simulink library "vmc"  (R2021b)
settings: Solver=VariableStepAuto  StartTime=0.0  StopTime=10.0  RelTol=1e-3
undefined symbols (not defined in the file or in its folder): AVMC_ACCDeltaTqIGain4OVRD_X_kph, AVMC_ACCDeltaTqIGain4OVRD_Y_mps2, AVMC_ACCDeltaTqIGain_X_kph, AVMC_ACCDeltaTqIGain_Y_mps2, AVMC_ACCDeltaTqPGain_X_kph, AVMC_ACCDeltaTqPGain_Y_kph, AVMC_ACCLongSteadyCtrl_X_kph, AVMC_ADSPosGFBDeltaTq_X_kph, AVMC_ADSPosGFBDeltaTq_Y_mps2, AVMC_AggressJerkPCT4AT_X_kph, AVMC_AggressJerkPCT_X_kph, AVMC_AggressLimitPCT4AT_X_kph, AVMC_AggressLimitPCT_X_kph, AVMC_CCLongSteadyCtrl_X_kph, AVMC_DISCDeltaTqIGain_X_kph, AVMC_DISCDeltaTqIGain_Y_mps2, AVMC_DISCDeltaTqPGain_X_kph, AVMC_DISCDeltaTqPGain_Y_kph, AVMC_ESCRegenOut_X_kph, AVMC_ESCRegenOut_Y_Deg, AVMC_ESCRegenOutEnSpd_X_Deg, AVMC_ISOAccLimit_X_mps, AVMC_ISODecLimit_X_mps, AVMC_ISOJerk_X_mps, AVMC_LatESCRegenOut_X_kph, AVMC_LatESCRegenOut_Y_Deg, AVMC_LongAccDeadZone_X_kph, AVMC_LongAccFiltTsforP2_X_Gps, AVMC_MCPresBaseTq_X_bar, AVMC_MSALongSteadyCtrl_X_kph, AVMC_MSAPedalOvrd_X_kph, AVMC_MSASpdBand_X_kph, AVMC_MSATqDownEndTq_X_kph, AVMC_MSATqDownTime_X_kph, AVMC_OPDDisSlideRate_X_Deg, AVMC_OVRD2ActSR2FCMCMD_X_mps2, AVMC_PedalTqRWhlRatio_X_Nm, AVMC_PedalTqRWhlRatio_Y_gps, AVMC_PedalTqRWhlSlipGain_X_rat, AVMC_PedalTqRWhlSlipGain_Y_kph, AVMC_PedalTqRWhSTRGGain_X_deg, AVMC_PedalTqRWhSTRGGain_Y_kph, AVMC_RDCDetectTime_X_kph, AVMC_RDCDetectTime_Y_pct, AVMC_RDCEnSlideRate_X_Deg, AVMC_RearWhlTqRatio_X_Nm, AVMC_RearWhlTqRatio_Y_gps, AVMC_RearWhlTqSlipGain_X_rat, AVMC_RearWhlTqSlipGain_Y_kph, AVMC_RearWhlTqSTRGGain_X_deg, AVMC_RearWhlTqSTRGGain_Y_kph, AVMC_ReqBrkJoinDecSR_X_mps2, AVMC_SoftJerkPCT_X_kph, AVMC_SoftLimitPCT_X_kph, AVMC_StESCYaw_X_kph, AVMC_StESCYaw_Y_Deg, AVMC_StESCYawCom_X_kph, AVMC_StESCYawCom_Y_Gps, AVMC_TMSpdBaseTq_X_rpm, AVMC_VehHoldDecCtrlTime2_X_kph ... (+411)
libraries: hcu_lib x108, simulink x82, tqr x1, simulink_extras x1
(part 8 of 14)

== system vmc/VMC/VMC/APS function/Signal Rounting1 ==
  VINP_SCPSystemMode_enum : Inport
  VVMC_APSActive_flg : Inport  Port=2
  VVMC_ADASActive_flg : Inport  Port=3
  VTQD_GearActualPosn_enum : Inport  Port=4
  VVMC_CAASActive_flg : Inport  Port=5
  VTQD_APSStaSys_enum : Inport  Port=6
  VTQD_APSDecReqA_flg : Inport  Port=7
  VTQD_APSDecReq_mps2 : Inport  Port=8
  VTQD_APSReq_enum : Inport  Port=9
  VINP_APSStaSystem_enum : Inport  Port=10
  VINP_APSDecReqA_flg : Inport  Port=11
  VINP_APSDecReq_mps2 : Inport  Port=12
  VINP_APSReq_enum : Inport  Port=13
  VVMC_SetACCDisableAPS_flg : Inport  Port=14
  Signal Determination VINP_APSDecReqAtest_flg : Subsystem
  Signal Determination VINP_APSDecReqtest_mps2 : Subsystem
  Signal Determination VINP_APSReqtest_enum : Subsystem
  Signal Determination VINP_APSStaSystemtest_enum : Subsystem
  Switch{,1..3} (4 alike) : Switch  Criteria=u2 > Threshold
  VVMC_APSStaSys_enum : Outport
  VVMC_APSDecReqA_flg : Outport  Port=2
  VVMC_APSDecReq_mps2 : Outport  Port=3
  VVMC_APSReq_enum : Outport  Port=4
  wires:
  [VINP_SCPSystemMode_enum] -> Signal Determination VINP_APSDecReqtest_mps2/3(VINP_SCPSystemMode_enum)
  Signal Determination VINP_APSDecReqAtest_flg/1(SignalOutp) -> VVMC_APSDecReqA_flg/1  "VVMC_APSDecReqA_flg"
  Signal Determination VINP_APSReqtest_enum/1(SignalOutp) -> VVMC_APSReq_enum/1  "VVMC_APSReq_enum"
  [VINP_SCPSystemMode_enum] -> Signal Determination VINP_APSReqtest_enum/3(VINP_SCPSystemMode_enum)
  Signal Determination VINP_APSStaSystemtest_enum/1(SignalOutp) -> VVMC_APSStaSys_enum/1  "VVMC_APSStaSys_enum"
  [VINP_SCPSystemMode_enum] -> Signal Determination VINP_APSDecReqAtest_flg/3(VINP_SCPSystemMode_enum)
  Signal Determination VINP_APSDecReqtest_mps2/1(SignalOutp) -> VVMC_APSDecReq_mps2/1  "VVMC_APSDecReq_mps2"
  VINP_SCPSystemMode_enum/1 -> [VINP_SCPSystemMode_enum]
  VVMC_APSActive_flg/1 -> [VVMC_APSActive_flg]
  VVMC_ADASActive_flg/1 -> [VVMC_ADASActive_flg]
  [VVMC_APSActive_flg] -> Signal Determination VINP_APSStaSystemtest_enum/4(VVMC_APSActive_flg)
  [VVMC_ADASActive_flg] -> Signal Determination VINP_APSStaSystemtest_enum/5(VVMC_ADASActive_flg)
  [VVMC_APSActive_flg] -> Signal Determination VINP_APSDecReqAtest_flg/4(VVMC_APSActive_flg)
  [VVMC_ADASActive_flg] -> Signal Determination VINP_APSDecReqAtest_flg/5(VVMC_ADASActive_flg)
  [VVMC_APSActive_flg] -> Signal Determination VINP_APSDecReqtest_mps2/4(VVMC_APSActive_flg)
  [VVMC_ADASActive_flg] -> Signal Determination VINP_APSDecReqtest_mps2/5(VVMC_ADASActive_flg)
  [VVMC_APSActive_flg] -> Signal Determination VINP_APSReqtest_enum/4(VVMC_APSActive_flg)
  [VVMC_ADASActive_flg] -> Signal Determination VINP_APSReqtest_enum/5(VVMC_ADASActive_flg)
  VTQD_GearActualPosn_enum/1 -> [VTQD_GearActualPosn_enum]
  [VTQD_GearActualPosn_enum] -> Signal Determination VINP_APSStaSystemtest_enum/6(VTQD_GearActualPosn_enum)
  [VINP_SCPSystemMode_enum] -> Signal Determination VINP_APSStaSystemtest_enum/3(VINP_SCPSystemMode_enum)
  [VINP_APSReq_enum] -> Signal Determination VINP_APSReqtest_enum/1(SignalInput1)
  VVMC_CAASActive_flg/1 -> [VVMC_CAASActive_flg]
  [VVMC_CAASActive_flg] -> Signal Determination VINP_APSStaSystemtest_enum/7(VVMC_CAASActive_flg)
  [VVMC_CAASActive_flg] -> Signal Determination VINP_APSDecReqAtest_flg/6(VVMC_CAASActive_flg)
  [VVMC_CAASActive_flg] -> Signal Determination VINP_APSDecReqtest_mps2/6(VVMC_CAASActive_flg)
  [VVMC_CAASActive_flg] -> Signal Determination VINP_APSReqtest_enum/6(VVMC_CAASActive_flg)
  VTQD_APSDecReq_mps2/1 -> [VTQD_APSDecReq_mps2]
  VTQD_APSReq_enum/1 -> [VTQD_APSReq_enum]
  VTQD_APSDecReqA_flg/1 -> [VTQD_APSDecReqA_flg]
  VTQD_APSStaSys_enum/1 -> [VTQD_APSStaSys_enum]
  Switch/1 -> Signal Determination VINP_APSStaSystemtest_enum/2(SignalInput2)
  Switch1/1 -> Signal Determination VINP_APSDecReqAtest_flg/2(SignalInput2)
  Switch2/1 -> Signal Determination VINP_APSDecReqtest_mps2/2(SignalInput2)
  Switch3/1 -> Signal Determination VINP_APSReqtest_enum/2(SignalInput2)
  VINP_APSStaSystem_enum/1 -> [VINP_APSStaSystem_enum]
  VINP_APSDecReqA_flg/1 -> [VINP_APSDecReqA_flg]
  VINP_APSReq_enum/1 -> [VINP_APSReq_enum]
  VINP_APSDecReq_mps2/1 -> [VINP_APSDecReq_mps2]
  [VINP_APSDecReq_mps2] -> Signal Determination VINP_APSDecReqtest_mps2/1(SignalInput1)
  [VINP_APSDecReqA_flg] -> Signal Determination VINP_APSDecReqAtest_flg/1(SignalInput1)
  [VINP_APSStaSystem_enum] -> Signal Determination VINP_APSStaSystemtest_enum/1(SignalInput1)
  VVMC_SetACCDisableAPS_flg/1 -> [VVMC_SetACCDisableAPS_flg]
  [VVMC_SetACCDisableAPS_flg] -> Switch/2
  [VINP_APSStaSystem_enum] -> Switch/1
  [VTQD_APSStaSys_enum] -> Switch/3
  [VVMC_SetACCDisableAPS_flg] -> Switch1/2
  [VTQD_APSDecReqA_flg] -> Switch1/3
  [VINP_APSDecReqA_flg] -> Switch1/1
  [VVMC_SetACCDisableAPS_flg] -> Switch2/2
  [VTQD_APSDecReq_mps2] -> Switch2/3
  [VINP_APSDecReq_mps2] -> Switch2/1
  [VVMC_SetACCDisableAPS_flg] -> Switch3/2
  [VTQD_APSReq_enum] -> Switch3/3
  [VINP_APSReq_enum] -> Switch3/1

== system vmc/VMC/VMC/APS function/Subsystem ==
  VINP_ADASACCSta_enum : Inport
  VINP_MCPressure_bar : Inport  Port=2
  VINP_BrkSwSta_flg : Inport  Port=3
  VINP_BrkPedalPos_pct : Inport  Port=4
  VTQD_APSDecReqA_flg : Inport  Port=5
  VINP_ACCObjDist_m : Inport  Port=6
  VVMC_MeterIndSpeedForCalcu_kph : Inport  Port=7
  VINP_VehSpeed_kph : Inport  Port=8
  0 : Constant  Value=KVMC_AllowSetSpdOvrd_flg
  1 : Constant  Value=KVMC_AllowSetSpdOvrdVal_flg
  2m : Constant  Value=KVMC_NotAllowSetSpdDist_m
  6m : Constant  Value=KVMC_AllowSetSpdDist_m
  AND : Logic  Inputs=6  AllPortsSameDT=off  OutDataTypeStr=boolean
  AND1 : Logic  Operator=OR  AllPortsSameDT=off  OutDataTypeStr=boolean
  AND3 : Logic  AllPortsSameDT=off  OutDataTypeStr=boolean
  Constant1 : Constant  Value=ENUM_ADASACCSTA_ACTIVE
  Constant2 : Constant  Value=ENUM_ADASACCSTA_STANDBY
  Constant4 : Constant  Value=KVMC_APSAllowSetACCMCP_bar
  Constant5 : Constant  Value=ZERO_FLOAT
  Constant6 : Constant  Value=TRUE
  Constant7 : Constant  Value=KVMC_APSAllowSetACCPosn_pct
  NOT : Logic  Operator=NOT  AllPortsSameDT=off  OutDataTypeStr=boolean
  NOT1 : Logic  Operator=NOT  AllPortsSameDT=off  OutDataTypeStr=boolean
  Relational Operator : RelationalOperator  Operator===  OutDataTypeStr=boolean  RndMeth=Simplest
  Relational Operator1 : RelationalOperator  Operator===  OutDataTypeStr=boolean  RndMeth=Simplest
  Relational Operator{2..4,6} (4 alike) : RelationalOperator  Operator=>  OutDataTypeStr=boolean  RndMeth=Simplest
  Relational Operator5 : RelationalOperator  Operator=<=  OutDataTypeStr=boolean  RndMeth=Simplest
  SR_Latch2 : hcu_lib/Basic_Blocks/SR_Latch
  Switch : Switch  Criteria=u2 > Threshold
  Switch1 : Switch  Criteria=u2 > Threshold
  VVMC_SetACCDisableAPS_flg : Outport
  wires:
  NOT1/1 -> AND/6
  Constant6/1 -> Switch/3
  Relational Operator4/1 -> AND/5
  AND/1 -> SR_Latch2/1
  Relational Operator1/1 -> AND1/1
  Constant2/1 -> Relational Operator/2
  Relational Operator3/1 -> NOT1/1
  Constant5/1 -> Relational Operator3/2
  Relational Operator/1 -> AND/1
  AND1/1 -> SR_Latch2/2
  Switch/1 -> VVMC_SetACCDisableAPS_flg/1  "VVMC_SetACCDisableAPS_flg"
  [VINP_VehSpeed_kph] -> Relational Operator3/1
  [VINP_MCPressure_bar] -> Relational Operator2/1
  [VVMC_AllowSetSpd_flg] -> AND/2
  [VINP_BrkSwSta_flg] -> NOT/1
  VINP_BrkSwSta_flg/1 -> [VINP_BrkSwSta_flg]
  NOT/1 -> AND1/2
  Constant7/1 -> Relational Operator4/2
  Constant4/1 -> Relational Operator2/2
  [VINP_BrkPedalPos_pct] -> Relational Operator4/1
  Constant1/1 -> Relational Operator1/2
  [VINP_ADASACCSta_enum] -> Relational Operator1/1
  [VINP_ADASACCSta_enum] -> Relational Operator/1
  SR_Latch2/1 -> Switch/1
  Relational Operator2/1 -> AND/4
  6m/1 -> Relational Operator5/2
  Relational Operator6/1 -> AND3/2
  1/1 -> Switch1/1
  [VINP_ACCObjDist_m] -> Relational Operator6/1, Relational Operator5/1
  2m/1 -> Relational Operator6/2
  Relational Operator5/1 -> AND3/1
  0/1 -> Switch1/2
  Switch1/1 -> [VVMC_AllowSetSpd_flg]  "VVMC_AllowSetSpd_flg"
  AND3/1 -> Switch1/3
  VINP_ACCObjDist_m/1 -> [VINP_ACCObjDist_m]
  VVMC_MeterIndSpeedForCalcu_kph/1 -> [VVMC_MeterIndSpeedForCalcu_kph]
  VINP_ADASACCSta_enum/1 -> [VINP_ADASACCSta_enum]
  VINP_MCPressure_bar/1 -> [VINP_MCPressure_bar]
  VINP_BrkPedalPos_pct/1 -> [VINP_BrkPedalPos_pct]
  [VINP_BrkSwSta_flg] -> AND/3
  VTQD_APSDecReqA_flg/1 -> [VTQD_APSDecReqA_flg]
  [VTQD_APSDecReqA_flg] -> Switch/2
  VINP_VehSpeed_kph/1 -> [VINP_VehSpeed_kph]

== system vmc/VMC/VMC/CruiseControlFunction/CCActiveDetermination ==
  VTQD_SpdCtrlMode_enum : Inport
  VVMC_FeatArbitrFinal_enum : Inport  Port=2
  VTQD_ExternalTqAllow_flg : Inport  Port=3
  VTQD_SWC1SetdownSta_flg : Inport  Port=4
  VTQD_SWC1ResUpSta_flg : Inport  Port=5
  VINP_VehSpeed_kph : Inport  Port=6
  VVMC_FeatSetSpdFinal_raw32 : Inport  Port=7
  VINP_BrakeSWGPIO_flg : Inport  Port=8
  VTQD_SWC1CANCELSta_flg : Inport  Port=9
  VINP_BrkSwSta_flg : Inport  Port=10
  VINP_ADASAEBSta_enum : Inport  Port=11
  VVMC_CCPedalOvrd_flg : Inport  Port=12
  VTQD_GearActualPosn_enum : Inport  Port=13
  VINP_Distanceunit_flg : Inport  Port=14
  VTQD_ExtDoorAllow_flg : Inport  Port=15
  VVMC_VMCCCCtrlAvail_flg : Inport  Port=16
  " 1" : Constant  Value=KTQD_CCActiveMetSpdLo_kph
  " 2" : Constant  Value=KTQD_CCActiveMetSpdLoMPH_mph
  3 : Constant  Value=KTQD_CCActiveMetSpdHi_kph
  5 : Constant  Value=KTQD_CCActiveMetSpdHiMPH_mph
  AND : Logic  AllPortsSameDT=off  OutDataTypeStr=boolean
  Cast To Single : DataTypeConversion  OutDataTypeStr=uint8
  Cast To Single1 : DataTypeConversion  OutDataTypeStr=boolean
  Cast To Single2 : DataTypeConversion  OutDataTypeStr=boolean
  Cast To Single3 : DataTypeConversion  OutDataTypeStr=single
  Cast To Single4 : DataTypeConversion  OutDataTypeStr=single
  Chart : Stateflow chart  TreatAsAtomicUnit=on
  Constant2 : Constant  Value=KVMC_CCMSASpdWar_kph
  Constant3 : Constant  Value=ENUM_FEATARBITRSTA_CC
  Constant4 : Constant  Value=TRUE
  Constant5 : Constant  Value=FALSE
  Constant6 : Constant  Value=ENUM_CCCRLSTA_ACTIVE
  Constant7 : Constant  Value=ENUM_ADASAEBSTA_ACTIVE
  Constant8 : Constant  Value=ENUM_GEARACTUALPOSN_D
  Delay : Delay  DelayLength=1
  Detect Decrease : simulink/Logic and Bit Operations/Detect Decrease  vinit=0.0  OutDataTypeStr=boolean
  Detect Decrease1 : simulink/Logic and Bit Operations/Detect Decrease  vinit=0.0  OutDataTypeStr=boolean
  Detect Decrease2 : simulink/Logic and Bit Operations/Detect Decrease  vinit=0.0  OutDataTypeStr=boolean
  Relational Operator : RelationalOperator  Operator===  OutDataTypeStr=boolean  RndMeth=Simplest
  Relational Operator1 : RelationalOperator  Operator===  OutDataTypeStr=boolean  RndMeth=Simplest
  Switch2 : Switch  Criteria=u2 > Threshold
  Switch3 : Switch  Criteria=u2 > Threshold
  u2 > 0 : Switch  Criteria=u2 > Threshold
  VVMC_CCCtrlSta_enum : Outport
  VVMC_CCSpdWar_flg : Outport  Port=2
  VVMC_CruzActive_flg : Outport  Port=3
  wires:
  Delay/1 -> Chart/15(VVMC_CCPedalOvrd_flg)
  [VVMC_CCPedalOvrd_flg] -> Delay/1
  VVMC_CCPedalOvrd_flg/1 -> [VVMC_CCPedalOvrd_flg]
  Constant7/1 -> Chart/14(ENUM_ADASAEBSTA_ACTIVE)
  [VINP_ADASAEBSta_enum] -> Chart/13(VINP_ADASAEBSta_enum)
  VINP_ADASAEBSta_enum/1 -> [VINP_ADASAEBSta_enum]
  Relational Operator1/1 -> AND/2
  Relational Operator/1 -> AND/1
  [VVMC_CCCtrlSta_enum] -> Relational Operator1/1
  Constant6/1 -> Relational Operator1/2
  Constant5/1 -> u2 > 0/3
  Constant4/1 -> u2 > 0/1
  AND/1 -> u2 > 0/2
  [VTQD_SpdCtrlMode_enum] -> Chart/1(VTQD_SpdCtrlMode_enum)
  VTQD_SpdCtrlMode_enum/1 -> [VTQD_SpdCtrlMode_enum]
  Constant3/1 -> Relational Operator/2
  Switch2/1 -> Cast To Single3/1
  [VINP_VehSpeed_kph] -> Chart/5(VINP_VehSpeed_kph)
  Switch3/1 -> Cast To Single4/1
  [VTQD_SWC1SetdownSta_flg] -> Detect Decrease/1
  [VVMC_FeatSetSpdFinal_raw32] -> Chart/7(VVMC_FeatSetSpdFinal_raw32)
  Constant2/1 -> Chart/8(KVMC_CCMSASpdWar_kph)
  [VTQD_ExternalTqAllow_flg] -> Chart/2(VTQD_ExternalTqAllow_flg)
  [VVMC_FeatArbitrFinal_enum] -> Relational Operator/1
  [VINP_BrakeSWGPIO_flg] -> Chart/9(VINP_BrakeSWGPIO_flg)
  [VTQD_SWC1CANCELSta_flg] -> Detect Decrease1/1
  [VTQD_SWC1ResUpSta_flg] -> Detect Decrease2/1
  Chart/1(VVMC_CCCtrlSta_enum) -> Cast To Single/1
  Chart/2(VVMC_CCSpdWar_flg) -> Cast To Single1/1
  u2 > 0/1 -> Cast To Single2/1
  VVMC_FeatArbitrFinal_enum/1 -> [VVMC_FeatArbitrFinal_enum]
  VTQD_ExternalTqAllow_flg/1 -> [VTQD_ExternalTqAllow_flg]
  VTQD_SWC1SetdownSta_flg/1 -> [VTQD_SWC1SetdownSta_flg]
  VTQD_SWC1ResUpSta_flg/1 -> [VTQD_SWC1ResUpSta_flg]
  VINP_VehSpeed_kph/1 -> [VINP_VehSpeed_kph]
  VVMC_FeatSetSpdFinal_raw32/1 -> [VVMC_FeatSetSpdFinal_raw32]
  VINP_BrakeSWGPIO_flg/1 -> [VINP_BrakeSWGPIO_flg]
  VTQD_SWC1CANCELSta_flg/1 -> [VTQD_SWC1CANCELSta_flg]
  VINP_BrkSwSta_flg/1 -> [VINP_BrkSwSta_flg]
  [VVMC_CCCtrlSta_enum] -> VVMC_CCCtrlSta_enum/1
  [VVMC_CCSpdWar_flg] -> VVMC_CCSpdWar_flg/1
  [VVMC_CruzActive_flg] -> VVMC_CruzActive_flg/1
  Detect Decrease/1 -> Chart/3(VVMC_DetectSWCSetDown_flg)  "VVMC_DetectSWCSetDown_flg"
  Detect Decrease1/1 -> Chart/10(VVMC_DetectSWCCANCEL_flg)  "VVMC_DetectSWCCANCEL_flg"
  Detect Decrease2/1 -> Chart/12(VVMC_DetectSWCResUp_flg)  "VVMC_DetectSWCResUp_flg"
  Cast To Single1/1 -> [VVMC_CCSpdWar_flg]  "VVMC_CCSpdWar_flg"
  Cast To Single2/1 -> [VVMC_CruzActive_flg]  "VVMC_CruzActive_flg"
  Cast To Single/1 -> [VVMC_CCCtrlSta_enum]  "VVMC_CCCtrlSta_enum"
  [VINP_BrkSwSta_flg] -> Chart/11(VINP_BrkSwSta_flg)
  VTQD_GearActualPosn_enum/1 -> [VTQD_GearActualPosn_enum]
  [VTQD_GearActualPosn_enum] -> Chart/16(VTQD_GearActualPosn_enum)
  Constant8/1 -> Chart/17(ENUM_GEARACTUALPOSN_D)
  3/1 -> Switch2/3
  5/1 -> Switch2/1
  [VINP_Distanceunit_flg] -> Switch2/2
  " 2"/1 -> Switch3/1
  [VINP_Distanceunit_flg] -> Switch3/2
  " 1"/1 -> Switch3/3
  VINP_Distanceunit_flg/1 -> [VINP_Distanceunit_flg]
  Cast To Single3/1 -> Chart/4(KVMC_CCActiveMetSpdHi_kph)
  Cast To Single4/1 -> Chart/6(KVMC_CCActiveMetSpdLo_kph)
  VTQD_ExtDoorAllow_flg/1 -> [VTQD_ExtDoorAllow_flg]
  [VTQD_ExtDoorAllow_flg] -> Chart/18(VTQD_ExtDoorAllow_flg)
  VVMC_VMCCCCtrlAvail_flg/1 -> [VVMC_VMCCCCtrlAvail_flg]
  [VVMC_VMCCCCtrlAvail_flg] -> Chart/19(VVMC_VMCCCCtrlAvail_flg)

== system vmc/VMC/VMC/CruiseControlFunction/CCDemandTorqueCalculation ==
  VVMC_FeatSetSpdForCalcu_kph : Inport
  VINP_VehSpeed_kph : Inport  Port=2
  VVMC_CruzActive_flg : Inport  Port=3
  VVMC_LongAcc_Gps : Inport  Port=4
  VVMC_CCPedalOvrd_flg : Inport  Port=5
  VVMC_ActACCRequiredAccel_mps2 : Inport  Port=6
  VVMC_SafetyCtrl_flg : Inport  Port=7
  VTQR_FrTMTqReq_Nm : Inport  Port=8
  VTQR_RrTMTqReq_Nm : Inport  Port=9
  VVMC_TotalAvailBrkRgnTq_Nm : Inport  Port=10
  AND12 : Logic  AllPortsSameDT=off  OutDataTypeStr=boolean
  Abs3 : Abs
  Abs4 : Abs
  Add{8,12,16,20..21} (5 alike) : Sum
  Add22 : Sum  Inputs=+-
  Add23 : Sum  Inputs=+-
  Cast To Single4 : DataTypeConversion  OutDataTypeStr=single
  Cast To Single5 : DataTypeConversion  OutDataTypeStr=single
  Constant1 : Constant  Value=KVMC_CCTqUpLim_Nm
  Constant104 : Constant  Value=ZERO_FLOAT
  Constant105 : Constant  Value=KTQD_RrTMTotalGearRatio_gain
  Constant106 : Constant  Value=KTQR_RrTMGearEff_c
  Constant107 : Constant  Value=KVMC_GravityValue_mps2
  Constant2 : Constant  Value=KVMC_CCTqLowLim_Nm
  Constant3 : Constant  Value=ZERO_FLOAT
  Constant36 : Constant  Value=KVMC_AccDevLowLim_mps2
  Constant38 : Constant  Value=KVMC_AccDevUpLim_mps2
  Constant4 : Constant  Value=KVMC_CCDISCPGainSW_flg
  Constant40 : Constant  Value=KVMC_CCSpdDevUpLim_kph
  Constant5 : Constant  Value=KVMC_CCTqUpLim_Nm
  Constant56 : Constant  Value=KVMC_CCSpdDevLowLim_kph
  Constant58 : Constant  Value=KVMC_Veh2MeterSpdFactor_enum
  Constant59 : Constant  Value=KVMC_Veh2MeterSpdOffset_enum
  Constant6 : Constant  Value=KVMC_CCTqLowLim_Nm
  Constant64 : Constant  Value=KVMC_TqSafetyCtrl_flg
  Constant65 : Constant  Value=KVMC_Veh2MeterSpdLoFactor_enum
  Constant7 : Constant  Value=ZERO_FLOAT
  Constant71 : Constant  Value=KTQR_FrTMGearEff_c
  Constant76 : Constant  Value=KTQD_FrTMTotalGearRatio_gain
  Data Type Conversion1 : DataTypeConversion  OutDataTypeStr=single
  Detect Decrease3 : simulink/Logic and Bit Operations/Detect Decrease  vinit=0.0  OutDataTypeStr=boolean
  Detect Increase3 : simulink/Logic and Bit Operations/Detect Increase  vinit=0.0  OutDataTypeStr=boolean
  Divide11 : Product  Inputs=**
  Divide12 : Product  Inputs=**
  Divide4 : Product  Inputs=***
  Divide7 : Product  Inputs=***
  InitialCondition: 1 : UnitDelay  SampleTime=-1  HasFrameUpgradeWarning=on
  Logical Operator1 : Logic  Operator=OR  AllPortsSameDT=off  OutDataTypeStr=boolean
  MVMC_DISCDeltaTqIGain_Z_Nm : Lookup_n-D  BreakpointsForDimension1=AVMC_DISCDeltaTqIGain_Y_mps2  BreakpointsForDimension2=AVMC_DISCDeltaTqIGain_X_kph  Table=MVMC_DISCDeltaTqIGain_Z_Nm  InternalRulePriority=Speed  RndMeth=Simplest  InputSameDT=on
      settings: InputPortMap=u0,u1
  MVMC_DISCDeltaTqPGain_Z_Nm : Lookup_n-D  BreakpointsForDimension1=AVMC_DISCDeltaTqPGain_Y_kph  BreakpointsForDimension2=AVMC_DISCDeltaTqPGain_X_kph  BreakpointsForDimension3=[5, 7]  Table=MVMC_DISCDeltaTqPGain_Z_Nm  ExtrapMethod=Clip  InternalRulePriority=Speed  RndMeth=Simplest  InputSameDT=on
      settings: InputPortMap=u0,u1
  Max : MinMax  Function=max  Inputs=2
  Max1 : MinMax  Function=max  Inputs=2
  Product2 : Product
  Relational Operator18 : RelationalOperator  Operator=<=  OutDataTypeStr=boolean  RndMeth=Simplest
  Saturation Dynamic{1,7..9} (4 alike) : simulink/Discontinuities/Saturation Dynamic  OutMin=[]  OutMax=[]  OutDataTypeStr=Inherit: Same as second input  OutDataType=fixdt(1, 16)  OutScaling=2^-10  DoSatur=off
  Switch{,2,5,7} (4 alike) : Switch  Criteria=u2 > Threshold
  Switch1 : Switch  Criteria=u2 > Threshold  Threshold=KVMC_Veh2MeterSpdLoBdy_kph
  Unit Delay3 : UnitDelay  SampleTime=-1  HasFrameUpgradeWarning=on
  u2 > 0 (3)1 : Switch  Criteria=u2 > Threshold
  u2 > 0 (4)1 : Switch  Criteria=u2 > Threshold
  VVMC_CruzWhlTqCal_Nm : Outport
  wires:
  VVMC_FeatSetSpdForCalcu_kph/1 -> [VVMC_FeatSetSpdForCalcu_kph]
  VVMC_CruzActive_flg/1 -> [VVMC_CruzActive_flg]
  VINP_VehSpeed_kph/1 -> [VINP_VehSpeed_kph]
  [VVMC_CruzWhlTqCal_Nm] -> VVMC_CruzWhlTqCal_Nm/1
  VVMC_LongAcc_Gps/1 -> [VVMC_LongAcc_Gps]
  VVMC_CCPedalOvrd_flg/1 -> [VVMC_CCPedalOvrd_flg]
  VVMC_ActACCRequiredAccel_mps2/1 -> [VVMC_CCReqAcc_mps2]
  VVMC_SafetyCtrl_flg/1 -> [VVMC_SafetyCtrl_flg]
  Switch5/1 -> Cast To Single5/1
  Detect Decrease3/1 -> Logical Operator1/2
  Divide4/1 -> Add16/1
  [VVMC_CruzActive_flg] -> Detect Increase3/1
  [VVMC_FeatSetSpdForCalcu_kph] -> MVMC_DISCDeltaTqPGain_Z_Nm/2
  Data Type Conversion1/1 -> Add23/1
  u2 > 0 (3)1/1 -> Switch5/1
  Constant71/1 -> Divide4/3
  Constant106/1 -> Divide7/3
  [VVMC_SafetyCtrl_flg] -> AND12/2
  Saturation Dynamic9/1 -> MVMC_DISCDeltaTqPGain_Z_Nm/1
  Relational Operator18/1 -> u2 > 0 (4)1/2
  [VVMC_LastCCWhlTqCalW_Nm] -> Abs3/1, u2 > 0 (4)1/1
  u2 > 0 (4)1/1 -> u2 > 0 (3)1/1  "VVMC_CruzWhlTqCalAftSafety_Nm"
  [VTQR_RrTMTqReq_Nm] -> Divide7/1
  [VVMC_LastCCWhlTqCalW_Nm] -> Add12/1
  MVMC_DISCDeltaTqIGain_Z_Nm/1 -> [VVMC_CCIGainDeltaTq_Nm]  "VVMC_CCIGainDeltaTq_Nm"
  Add23/1 -> Saturation Dynamic9/2
  Constant104/1 -> Switch5/3
  InitialCondition: 1/1 -> [VVMC_LastCCWhlTqCalW_Nm]  "VVMC_LastCruzWhlTqCal_Nm"
  Detect Increase3/1 -> Logical Operator1/1
  [VINP_VehSpeed_kph] -> MVMC_DISCDeltaTqIGain_Z_Nm/2
  [VVMC_CCIGainDeltaTq_Nm] -> Add12/2
  Abs4/1 -> Relational Operator18/2
  Saturation Dynamic7/1 -> InitialCondition: 1/1, Add21/2
  Abs3/1 -> Relational Operator18/1
  [VTQR_FrTMTqReq_Nm] -> Divide4/1
  Saturation Dynamic8/1 -> MVMC_DISCDeltaTqIGain_Z_Nm/1
  [VVMC_CCIGainDeltaTq_Nm] -> Add20/2
  Constant76/1 -> Divide4/2
  Divide7/1 -> Add16/2
  AND12/1 -> u2 > 0 (3)1/2
  Add20/1 -> Switch7/1
  Constant105/1 -> Divide7/2
  [VVMC_CruzActive_flg] -> Switch5/2
  [VVMC_CCPedalOvrd_flg] -> Unit Delay3/1
  Cast To Single5/1 -> Saturation Dynamic7/2
  Switch7/1 -> Cast To Single4/1
  Add12/1 -> Switch7/3
  Constant40/1 -> Saturation Dynamic9/1
  Constant5/1 -> Saturation Dynamic7/1
  Add16/1 -> Add20/1
  Unit Delay3/1 -> Detect Decrease3/1
  [VVMC_CCReqAcc_mps2] -> Add22/1
  Add22/1 -> Saturation Dynamic8/2
  Constant107/1 -> Product2/2
  Constant64/1 -> AND12/1
  [VVMC_FeatSetSpdForCalcu_kph] -> Data Type Conversion1/1
  Logical Operator1/1 -> Switch7/2
  Constant38/1 -> Saturation Dynamic8/1
  Product2/1 -> Add22/2
  [VVMC_LongAcc_Gps] -> Product2/1
  Constant36/1 -> Saturation Dynamic8/3
  Constant6/1 -> Max/1
  Constant56/1 -> Saturation Dynamic9/3
  Cast To Single4/1 -> u2 > 0 (4)1/3, Abs4/1, u2 > 0 (3)1/3
  VTQR_FrTMTqReq_Nm/1 -> [VTQR_FrTMTqReq_Nm]
  VTQR_RrTMTqReq_Nm/1 -> [VTQR_RrTMTqReq_Nm]
  VVMC_TotalAvailBrkRgnTq_Nm/1 -> [VVMC_TotalAvailBrkRgnTq_Nm]
  [VVMC_TotalAvailBrkRgnTq_Nm] -> Max/2
  Max/1 -> Saturation Dynamic7/3
  Switch/1 -> [VVMC_CCPGainDeltaTq_Nm]  "VVMC_CCPGainDeltaTq_Nm"
  Switch2/1 -> Add21/1
  [VVMC_CCPGainDeltaTq_Nm] -> Switch2/1
  Constant4/1 -> Switch2/2
  Constant7/1 -> Switch2/3
  Saturation Dynamic1/1 -> [VVMC_CruzWhlTqCal_Nm]  "VVMC_CruzWhlTqCal_Nm"
  [VINP_VehSpeed_kph] -> Divide11/2, Switch1/2, Divide12/1
  Switch1/1 -> Add23/2
  Constant59/1 -> Add8/1
  Add8/1 -> Switch1/1
  Constant58/1 -> Divide11/1
  Constant65/1 -> Divide12/2
  Divide11/1 -> Add8/2
  Divide12/1 -> Switch1/3
  Max1/1 -> Saturation Dynamic1/3
  [VVMC_TotalAvailBrkRgnTq_Nm] -> Max1/2
  Constant2/1 -> Max1/1
  Constant1/1 -> Saturation Dynamic1/1
  Add21/1 -> Saturation Dynamic1/2
  [VVMC_CruzActive_flg] -> Switch/2
  MVMC_DISCDeltaTqPGain_Z_Nm/1 -> Switch/1
  Constant3/1 -> Switch/3

== system vmc/VMC/VMC/CruiseControlFunction/CCTorqueSourceDetermination ==
  VTQD_DriverWhlTqDem_Nm : Inport
  VVMC_CruzWhlTqCal_Nm : Inport  Port=2
  VTQD_LowIdleAccPedal_flg : Inport  Port=3
  VTQD_RegenMode_enum : Inport  Port=4
  VVMC_FeatArbitrFinal_enum : Inport  Port=5
  task_time_s : Inport  Port=6
  AND1 : Logic  Inputs=3  AllPortsSameDT=off  OutDataTypeStr=boolean
  Add : Sum
  Constant20 : Constant  Value=FALSE
  Constant21 : Constant  Value=ENUM_FEATARBITRSTA_CC
  Constant22 : Constant  Value=TRUE
  Constant23 : Constant  Value=KVMC_ACCPedalOvrdRestTime_s
  DelayEnable : hcu_lib/Basic_Blocks/DelayEnable
  Direct Lookup Table (n-D)1 : LookupNDDirect  NumberOfTableDimensions=1  Table=MVMC_ACCPedalOvrdTqHys_Y_Nm
  NOT2 : Logic  Operator=NOT  AllPortsSameDT=off  OutDataTypeStr=boolean
  OR1 : Logic  Operator=OR  AllPortsSameDT=off  OutDataTypeStr=boolean
  Relational Operator6 : RelationalOperator  Operator===  OutDataTypeStr=boolean  RndMeth=Simplest
  Relational Operator7 : RelationalOperator  Operator=>  OutDataTypeStr=boolean  RndMeth=Simplest
  Relational Operator8 : RelationalOperator  Operator=<=  OutDataTypeStr=boolean  RndMeth=Simplest
  SR_Latch : hcu_lib/Basic_Blocks/SR_Latch
  u2 > 0 (1) : Switch  Criteria=u2 > Threshold
  u2 > 0 (2) : Switch  Criteria=u2 > Threshold
  VVMC_CruzWhlTqReq_Nm : Outport
  VVMC_CCPedalOvrd_flg : Outport  Port=2
  wires:
  VTQD_DriverWhlTqDem_Nm/1 -> [VTQD_DriverWhlTqDem_Nm]
  VVMC_CruzWhlTqCal_Nm/1 -> [VVMC_CruzWhlTqCal_Nm]
  [VVMC_CruzWhlTqReq_Nm] -> VVMC_CruzWhlTqReq_Nm/1
  VTQD_LowIdleAccPedal_flg/1 -> [VTQD_LowIdleAccPedal_flg]
  [VVMC_CCPedalOvrd_flg] -> VVMC_CCPedalOvrd_flg/1
  [task_time_s] -> DelayEnable/3
  [VTQD_LowIdleAccPedal_flg] -> NOT2/1
  [VTQD_DriverWhlTqDem_Nm] -> u2 > 0 (1)/1
  [VVMC_CruzWhlTqCal_Nm] -> u2 > 0 (1)/3
  [VVMC_CruzWhlTqCal_Nm] -> Relational Operator8/2
  [VVMC_CruzWhlTqCal_Nm] -> Add/1
  u2 > 0 (2)/1 -> [VVMC_CCPedalOvrd_flg]
  Add/1 -> Relational Operator7/2
  [VTQD_DriverWhlTqDem_Nm] -> Relational Operator7/1
  [VVMC_FeatArbitrFinal_enum] -> Relational Operator6/1
  OR1/1 -> SR_Latch/2
  Relational Operator8/1 -> DelayEnable/1
  Constant23/1 -> DelayEnable/2
  u2 > 0 (1)/1 -> [VVMC_CruzWhlTqReq_Nm]
  Relational Operator7/1 -> SR_Latch/1
  [VVMC_CCPedalTqEnOvrd_flg] -> AND1/3
  NOT2/1 -> AND1/2
  Constant20/1 -> u2 > 0 (2)/3
  Relational Operator6/1 -> AND1/1
  [VTQD_RegenMode_enum] -> Direct Lookup Table (n-D)1/1
  [VTQD_DriverWhlTqDem_Nm] -> Relational Operator8/1
  DelayEnable/1 -> OR1/1
  SR_Latch/1 -> [VVMC_CCPedalTqEnOvrd_flg]  "VVMC_CCPedalTqEnOvrd_flg"
  [VTQD_LowIdleAccPedal_flg] -> OR1/2
  AND1/1 -> u2 > 0 (1)/2, u2 > 0 (2)/2
  Constant21/1 -> Relational Operator6/2
  Direct Lookup Table (n-D)1/1 -> Add/2
  Constant22/1 -> u2 > 0 (2)/1
  VTQD_RegenMode_enum/1 -> [VTQD_RegenMode_enum]
  VVMC_FeatArbitrFinal_enum/1 -> [VVMC_FeatArbitrFinal_enum]
  task_time_s/1 -> [task_time_s]

== system vmc/VMC/VMC/IMU/IMU memorized offset result ==
  VINP_MemOffsetGyroX_raw16 : Inport
  VINP_MemOffsetGyroY_raw16 : Inport  Port=2
  VINP_MemOffsetGyroZ_raw16 : Inport  Port=3
  VINP_MemOffsetAccX_raw16 : Inport  Port=4
  VINP_MemOffsetAccY_raw16 : Inport  Port=5
  VINP_MemOffsetAccZ_raw16 : Inport  Port=6
  ACCEL_FS_SEL = 001 SENSITIVITY = 2000 LSB/g : Constant  Value=KVMC_AccFSCalSet_enum
  Constant6 : Constant  Value=ONE_FLOAT  OutDataTypeStr=single
  Data Type Conversion : DataTypeConversion  OutDataTypeStr=uint16
  Data Type Conversion{1..6} (6 alike) : DataTypeConversion  OutDataTypeStr=single
  Data Type Conversion7 : DataTypeConversion  OutDataTypeStr=uint16
  Divide{,1..5} (6 alike) : Product  Inputs=**
  GYRO_FS_SEL = 0001 SENSITIVITY = 50 LSB/dps : Constant  Value=KVMC_GyroFSCalSet_enum
  Math Function{,1..5} (6 alike) : Math  Operator=reciprocal  SaturateOnIntegerOverflow=on
  Plus : Sum  Inputs=+-
  VVMC_MemOffsetGyroX_Dps : Outport
  VVMC_MemOffsetGyroY_Dps : Outport  Port=2
  VVMC_MemOffsetGyroZ_Dps : Outport  Port=3
  VVMC_MemOffsetAccX_G : Outport  Port=4
  VVMC_MemOffsetAccY_G : Outport  Port=5
  VVMC_MemOffsetAccZ_G : Outport  Port=6
  wires:
  VINP_MemOffsetGyroX_raw16/1 -> [VINP_MemOffsetGyroX_raw16]
  VINP_MemOffsetGyroY_raw16/1 -> [VINP_MemOffsetGyroY_raw16]
  [VINP_MemOffsetGyroX_raw16] -> Divide/1
  [VVMC_GyroFSCalSet_enum] -> Data Type Conversion1/1
  GYRO_FS_SEL = 0001 SENSITIVITY = 50 LSB/dps/1 -> Data Type Conversion/1
  Data Type Conversion/1 -> [VVMC_GyroFSCalSet_enum]  "VVMC_GyroFSCalSet_enum"
  [VVMC_GyroFSCalSet_enum] -> Data Type Conversion2/1
  [VINP_MemOffsetGyroY_raw16] -> Divide1/1
  [VINP_MemOffsetGyroZ_raw16] -> Divide2/1
  [VVMC_GyroFSCalSet_enum] -> Data Type Conversion3/1
  [VVMC_AccFSCalSet_enum] -> Data Type Conversion4/1
  [VINP_MemOffsetAccX_raw16] -> Divide3/1
  [VINP_MemOffsetAccY_raw16] -> Divide4/1
  [VVMC_AccFSCalSet_enum] -> Data Type Conversion5/1
  [VVMC_AccFSCalSet_enum] -> Data Type Conversion6/1
  [VINP_MemOffsetAccZ_raw16] -> Divide5/1
  Data Type Conversion7/1 -> [VVMC_AccFSCalSet_enum]  "VVMC_AccFSCalSet_enum"
  ACCEL_FS_SEL = 001 SENSITIVITY = 2000 LSB/g/1 -> Data Type Conversion7/1
  Divide/1 -> [VVMC_MemOffsetGyroX_Dps]  "VVMC_MemOffsetGyroX_Dps"
  Divide1/1 -> [VVMC_MemOffsetGyroY_Dps]  "VVMC_MemOffsetGyroY_Dps"
  Divide2/1 -> [VVMC_MemOffsetGyroZ_Dps]  "VVMC_MemOffsetGyroZ_Dps"
  Divide3/1 -> [VVMC_MemOffsetAccX_G]  "VVMC_MemOffsetAccX_G"
  Plus/1 -> [VVMC_MemOffsetAccZ_G]  "VVMC_MemOffsetAccZ_G"
  Divide5/1 -> Plus/1
  Constant6/1 -> Plus/2
  [VVMC_MemOffsetGyroX_Dps] -> VVMC_MemOffsetGyroX_Dps/1
  [VVMC_MemOffsetGyroY_Dps] -> VVMC_MemOffsetGyroY_Dps/1
  [VVMC_MemOffsetGyroZ_Dps] -> VVMC_MemOffsetGyroZ_Dps/1
  [VVMC_MemOffsetAccX_G] -> VVMC_MemOffsetAccX_G/1
  [VVMC_MemOffsetAccY_G] -> VVMC_MemOffsetAccY_G/1
  [VVMC_MemOffsetAccZ_G] -> VVMC_MemOffsetAccZ_G/1
  Divide4/1 -> [VVMC_MemOffsetAccY_G]  "VVMC_MemOffsetAccY_G"
  VINP_MemOffsetGyroZ_raw16/1 -> [VINP_MemOffsetGyroZ_raw16]
  VINP_MemOffsetAccX_raw16/1 -> [VINP_MemOffsetAccX_raw16]
  VINP_MemOffsetAccY_raw16/1 -> [VINP_MemOffsetAccY_raw16]
  VINP_MemOffsetAccZ_raw16/1 -> [VINP_MemOffsetAccZ_raw16]
  Math Function/1 -> Divide/2
  Math Function1/1 -> Divide1/2
  Math Function2/1 -> Divide2/2
  Math Function3/1 -> Divide3/2
  Math Function4/1 -> Divide4/2
  Math Function5/1 -> Divide5/2
  Data Type Conversion1/1 -> Math Function/1
  Data Type Conversion2/1 -> Math Function1/1
  Data Type Conversion3/1 -> Math Function2/1
  Data Type Conversion4/1 -> Math Function3/1
  Data Type Conversion5/1 -> Math Function4/1
  Data Type Conversion6/1 -> Math Function5/1

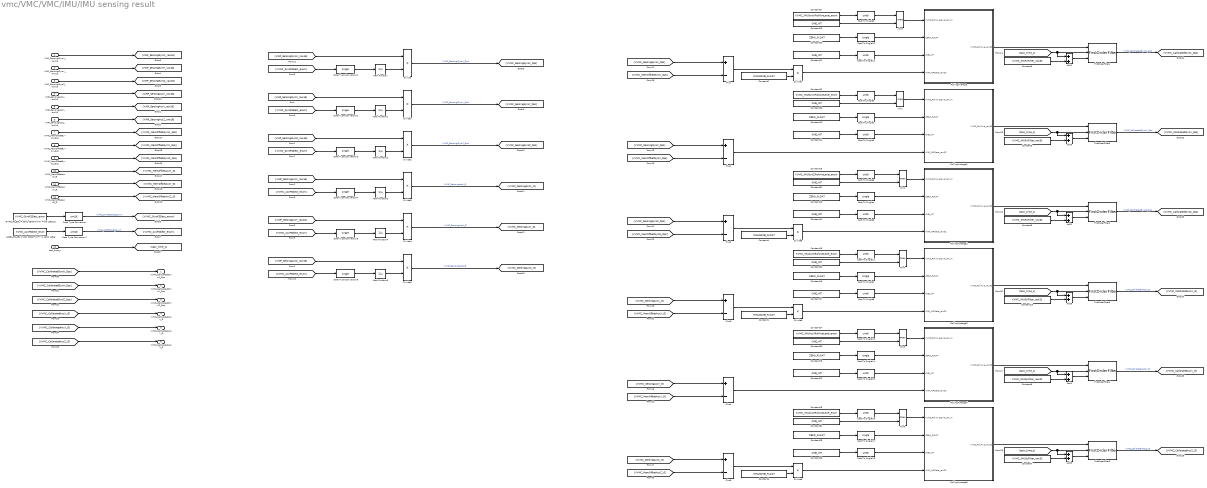
== system vmc/VMC/VMC/IMU/IMU sensing result  ==
  VINP_SensingGyroX_raw16 : Inport
  VINP_SensingGyroY_raw16 : Inport  Port=2
  VINP_SensingGyroZ_raw16 : Inport  Port=3
  VINP_SensingAccX_raw16 : Inport  Port=4
  VINP_SensingAccY_raw16 : Inport  Port=5
  VINP_SensingAccZ_raw16 : Inport  Port=6
  VVMC_MemOffsetGyroX_Dps : Inport  Port=7
  VVMC_MemOffsetGyroY_Dps : Inport  Port=8
  VVMC_MemOffsetGyroZ_Dps : Inport  Port=9
  VVMC_MemOffsetAccX_G : Inport  Port=10
  VVMC_MemOffsetAccY_G : Inport  Port=11
  VVMC_MemOffsetAccZ_G : Inport  Port=12
  task_time_s : Inport  Port=13
  ACCEL_FS_SEL = 001 SENSITIVITY = 2000 LSB/g : Constant  Value=KVMC_AccFSSlect_enum
  Add{1..5,8} (6 alike) : Sum
  Cast To Single{1,4,7,10,14,17} (6 alike) : DataTypeConversion  OutDataTypeStr=single
  Cast To Single{2..3,5..6,8..9,11..13,15..16,18} (12 alike) : DataTypeConversion  OutDataTypeStr=uint8
  Constant{1..2,4,6} (4 alike) : Constant  Value=MINUSONE_FLOAT
  Constant{10,13,16,19..20,25} (6 alike) : Constant  Value=ZERO_FLOAT
  Constant{11,14,17,21..22,26,29..34} (12 alike) : Constant  Value=ONE_INT
  Constant12 : Constant  Value=KVMC_IMUGyroYRollAveLevel_enum
  Constant15 : Constant  Value=KVMC_IMUGyroZRollAveLevel_enum
  Constant18 : Constant  Value=KVMC_IMUAccXRollAveLevel_enum
  Constant23 : Constant  Value=KVMC_IMUGxFilter_raw32
  Constant24 : Constant  Value=KVMC_IMUAccYRollAveLevel_enum
  Constant27 : Constant  Value=KVMC_IMUGyroXRollAveLevel_enum
  Constant28 : Constant  Value=KVMC_IMUAccZRollAveLevel_enum
  Constant3 : Constant  Value=KVMC_IMURxFilter_raw32
  Constant5 : Constant  Value=KVMC_IMURzFilter_raw32
  Constant7 : Constant  Value=KVMC_IMUGzFilter_raw32
  Constant8 : Constant  Value=KVMC_IMUGyFilter_raw32
  Constant9 : Constant  Value=KVMC_IMURyFilter_raw32
  Data Type Conversion : DataTypeConversion  OutDataTypeStr=uint16
  Data Type Conversion{1..6} (6 alike) : DataTypeConversion  OutDataTypeStr=single
  Data Type Conversion7 : DataTypeConversion  OutDataTypeStr=uint16
  Divide{,1..9} (10 alike) : Product  Inputs=**
  FirstOrderFilter{1..6} (6 alike) : hcu_lib/Basic_Blocks/FirstOrderFilter
  GYRO_FS_SEL = 0001 SENSITIVITY = 50 LSB/dps : Constant  Value=KVMC_GyroFSSlect_enum
  Math Function{,1..5} (6 alike) : Math  Operator=reciprocal  SaturateOnIntegerOverflow=on
  Min{1..6} (6 alike) : MinMax  Function=max  Inputs=2
  Plus{,1..5} (6 alike) : Sum  Inputs=+-
  RollingAverage : Stateflow chart  TreatAsAtomicUnit=on
  RollingAverage1 : Stateflow chart  TreatAsAtomicUnit=on
  RollingAverage2 : Stateflow chart  TreatAsAtomicUnit=on
  RollingAverage3 : Stateflow chart  TreatAsAtomicUnit=on
  RollingAverage4 : Stateflow chart  TreatAsAtomicUnit=on
  RollingAverage5 : Stateflow chart  TreatAsAtomicUnit=on
  VVMC_CalibratedGyroX_Dps : Outport
  VVMC_CalibratedGyroY_Dps : Outport  Port=2
  VVMC_CalibratedGyroZ_Dps : Outport  Port=3
  VVMC_CalibratedAccX_G : Outport  Port=4
  VVMC_CalibratedAccY_G : Outport  Port=5
  VVMC_CalibratedAccZ_G : Outport  Port=6
  wires:
  Divide4/1 -> [VVMC_SensingAccY_G]  "VVMC_SensingAccY_G"
  Divide3/1 -> [VVMC_SensingAccX_G]  "VVMC_SensingAccX_G"
  Divide2/1 -> [VVMC_SensingGyroZ_Dps]  "VVMC_SensingGyroZ_Dps"
  Divide1/1 -> [VVMC_SensingGyroY_Dps]  "VVMC_SensingGyroY_Dps"
  ACCEL_FS_SEL = 001 SENSITIVITY = 2000 LSB/g/1 -> Data Type Conversion7/1
  Data Type Conversion7/1 -> [VVMC_AccFSSlect_enum]  "VVMC_AccFSSlect_enum"
  [VINP_SensingAccZ_raw16] -> Divide5/1
  [VVMC_AccFSSlect_enum] -> Data Type Conversion5/1
  [VINP_SensingAccY_raw16] -> Divide4/1
  [VINP_SensingAccX_raw16] -> Divide3/1
  [VVMC_GyroFSSlect_enum] -> Data Type Conversion3/1
  [VINP_SensingGyroZ_raw16] -> Divide2/1
  [VINP_SensingGyroY_raw16] -> Divide1/1
  [VVMC_GyroFSSlect_enum] -> Data Type Conversion2/1
  Data Type Conversion/1 -> [VVMC_GyroFSSlect_enum]  "VVMC_GyroFSSlect_enum"
  GYRO_FS_SEL = 0001 SENSITIVITY = 50 LSB/dps/1 -> Data Type Conversion/1
  [VVMC_GyroFSSlect_enum] -> Data Type Conversion1/1
  [VINP_SensingGyroX_raw16] -> Divide/1
  VVMC_MemOffsetGyroY_Dps/1 -> [VVMC_MemOffsetGyroY_Dps]
  VVMC_MemOffsetGyroX_Dps/1 -> [VVMC_MemOffsetGyroX_Dps]
  VVMC_MemOffsetAccY_G/1 -> [VVMC_MemOffsetAccY_G]
  VVMC_MemOffsetAccZ_G/1 -> [VVMC_MemOffsetAccZ_G]
  VVMC_MemOffsetGyroZ_Dps/1 -> [VVMC_MemOffsetGyroZ_Dps]
  VVMC_MemOffsetAccX_G/1 -> [VVMC_MemOffsetAccX_G]
  VINP_SensingGyroX_raw16/1 -> [VINP_SensingGyroX_raw16]
  VINP_SensingGyroY_raw16/1 -> [VINP_SensingGyroY_raw16]
  VINP_SensingGyroZ_raw16/1 -> [VINP_SensingGyroZ_raw16]
  VINP_SensingAccX_raw16/1 -> [VINP_SensingAccX_raw16]
  VINP_SensingAccY_raw16/1 -> [VINP_SensingAccY_raw16]
  VINP_SensingAccZ_raw16/1 -> [VINP_SensingAccZ_raw16]
  Divide5/1 -> [VVMC_SensingAccZ_G]  "VVMC_SensingAccZ_G"
  Divide/1 -> [VVMC_SensingGyroX_Dps]  "VVMC_SensingGyroX_Dps"
  [VVMC_SensingGyroX_Dps] -> Plus/1
  [VVMC_MemOffsetGyroX_Dps] -> Plus/2
  [VVMC_SensingGyroY_Dps] -> Plus1/1
  [VVMC_MemOffsetGyroY_Dps] -> Plus1/2
  [VVMC_SensingGyroZ_Dps] -> Plus2/1
  [VVMC_MemOffsetGyroZ_Dps] -> Plus2/2
  [VVMC_SensingAccX_G] -> Plus3/1
  [VVMC_MemOffsetAccX_G] -> Plus3/2
  [VVMC_SensingAccY_G] -> Plus4/1
  [VVMC_MemOffsetAccY_G] -> Plus4/2
  [VVMC_SensingAccZ_G] -> Plus5/1
  [VVMC_MemOffsetAccZ_G] -> Plus5/2
  FirstOrderFilter1/1 -> [VVMC_CalibratedGyroX_Dps]  "VVMC_CalibratedGyroX_Dps"
  FirstOrderFilter5/1 -> [VVMC_CalibratedGyroY_Dps]  "VVMC_CalibratedGyroY_Dps"
  FirstOrderFilter2/1 -> [VVMC_CalibratedGyroZ_Dps]  "VVMC_CalibratedGyroZ_Dps"
  FirstOrderFilter6/1 -> [VVMC_CalibratedAccX_G]  "VVMC_CalibratedAccX_G"
  FirstOrderFilter4/1 -> [VVMC_CalibratedAccY_G]  "VVMC_CalibratedAccY_G"
  FirstOrderFilter3/1 -> [VVMC_CalibratedAccZ_G]  "VVMC_CalibratedAccZ_G"
  Math Function/1 -> Divide/2
  Math Function1/1 -> Divide1/2
  Math Function2/1 -> Divide2/2
  Math Function3/1 -> Divide3/2
  Math Function4/1 -> Divide4/2
  Math Function5/1 -> Divide5/2
  Data Type Conversion1/1 -> Math Function/1
  Data Type Conversion2/1 -> Math Function1/1
  Data Type Conversion3/1 -> Math Function2/1
  [VVMC_AccFSSlect_enum] -> Data Type Conversion4/1
  Data Type Conversion4/1 -> Math Function3/1
  Data Type Conversion5/1 -> Math Function4/1
  [VVMC_AccFSSlect_enum] -> Data Type Conversion6/1
  Data Type Conversion6/1 -> Math Function5/1
  task_time_s/1 -> [task_time_s]
  [task_time_s] -> Add8/1, FirstOrderFilter6/2
  Plus3/1 -> Divide6/1
  Constant23/1 -> Add8/2
  Add8/1 -> FirstOrderFilter6/3
  Constant1/1 -> Divide6/2
  Divide6/1 -> RollingAverage3/4(VINP_INPData_raw32)
  Divide7/1 -> RollingAverage/4(VINP_INPData_raw32)
  Constant2/1 -> Divide7/2
  Add1/1 -> FirstOrderFilter1/3
  Constant3/1 -> Add1/2
  [task_time_s] -> FirstOrderFilter1/2, Add1/1
  Plus/1 -> Divide7/1
  [task_time_s] -> Add2/1, FirstOrderFilter2/2
  Constant5/1 -> Add2/2
  Add2/1 -> FirstOrderFilter2/3
  Constant4/1 -> Divide8/2
  Divide8/1 -> RollingAverage2/4(VINP_INPData_raw32)
  Plus2/1 -> Divide8/1
  Divide9/1 -> RollingAverage5/4(VINP_INPData_raw32)
  Constant6/1 -> Divide9/2
  Add3/1 -> FirstOrderFilter3/3
  Constant7/1 -> Add3/2
  [task_time_s] -> FirstOrderFilter3/2, Add3/1
  Plus5/1 -> Divide9/1
  Add4/1 -> FirstOrderFilter4/3
  Constant8/1 -> Add4/2
  [task_time_s] -> FirstOrderFilter4/2, Add4/1
  Plus4/1 -> RollingAverage4/4(VINP_INPData_raw32)
  [task_time_s] -> Add5/1, FirstOrderFilter5/2
  Constant9/1 -> Add5/2
  Add5/1 -> FirstOrderFilter5/3
  Plus1/1 -> RollingAverage1/4(VINP_INPData_raw32)
  Constant20/1 -> Cast To Single10/1
  Constant27/1 -> Cast To Single9/1
  Cast To Single12/1 -> RollingAverage/3(ONE_INT)
  Cast To Single9/1 -> Min3/1
  Cast To Single10/1 -> RollingAverage/2(ZERO_FLOAT)
  Constant21/1 -> Cast To Single12/1
  RollingAverage/1(VVMC_RollAve_raw32) -> FirstOrderFilter1/1
  Constant11/1 -> Cast To Single2/1
  Cast To Single1/1 -> RollingAverage1/2(ZERO_FLOAT)
  Cast To Single3/1 -> Min1/1
  Cast To Single2/1 -> RollingAverage1/3(ONE_INT)
  Constant12/1 -> Cast To Single3/1
  Constant10/1 -> Cast To Single1/1
  RollingAverage1/1(VVMC_RollAve_raw32) -> FirstOrderFilter5/1
  Constant13/1 -> Cast To Single4/1
  Constant15/1 -> Cast To Single6/1
  Constant14/1 -> Cast To Single5/1
  Cast To Single6/1 -> Min2/1
  Cast To Single4/1 -> RollingAverage2/2(ZERO_FLOAT)
  Cast To Single5/1 -> RollingAverage2/3(ONE_INT)
  RollingAverage2/1(VVMC_RollAve_raw32) -> FirstOrderFilter2/1
  Constant17/1 -> Cast To Single8/1
  Cast To Single7/1 -> RollingAverage3/2(ZERO_FLOAT)
  Cast To Single11/1 -> Min4/1
  Cast To Single8/1 -> RollingAverage3/3(ONE_INT)
  Constant18/1 -> Cast To Single11/1
  Constant16/1 -> Cast To Single7/1
  RollingAverage3/1(VVMC_RollAve_raw32) -> FirstOrderFilter6/1
  Constant19/1 -> Cast To Single14/1
  Constant24/1 -> Cast To Single13/1
  Cast To Single15/1 -> RollingAverage4/3(ONE_INT)
  Cast To Single13/1 -> Min5/1
  Cast To Single14/1 -> RollingAverage4/2(ZERO_FLOAT)
  Constant22/1 -> Cast To Single15/1
  RollingAverage4/1(VVMC_RollAve_raw32) -> FirstOrderFilter4/1
  Constant26/1 -> Cast To Single18/1
  Cast To Single17/1 -> RollingAverage5/2(ZERO_FLOAT)
  Cast To Single16/1 -> Min6/1
  Cast To Single18/1 -> RollingAverage5/3(ONE_INT)
  Constant28/1 -> Cast To Single16/1
  Constant25/1 -> Cast To Single17/1
  RollingAverage5/1(VVMC_RollAve_raw32) -> FirstOrderFilter3/1
  [VVMC_CalibratedGyroX_Dps] -> VVMC_CalibratedGyroX_Dps/1
  [VVMC_CalibratedGyroY_Dps] -> VVMC_CalibratedGyroY_Dps/1
  [VVMC_CalibratedGyroZ_Dps] -> VVMC_CalibratedGyroZ_Dps/1
  [VVMC_CalibratedAccX_G] -> VVMC_CalibratedAccX_G/1
  [VVMC_CalibratedAccY_G] -> VVMC_CalibratedAccY_G/1
  [VVMC_CalibratedAccZ_G] -> VVMC_CalibratedAccZ_G/1
  Constant29/1 -> Min3/2
  Min3/1 -> RollingAverage/1(KVMC_RollAveLevel_enum)
  Constant30/1 -> Min1/2
  Min1/1 -> RollingAverage1/1(KVMC_RollAveLevel_enum)
  Constant31/1 -> Min2/2
  Min2/1 -> RollingAverage2/1(KVMC_RollAveLevel_enum)
  Constant32/1 -> Min4/2
  Min4/1 -> RollingAverage3/1(KVMC_RollAveLevel_enum)
  Constant33/1 -> Min5/2
  Min5/1 -> RollingAverage4/1(KVMC_RollAveLevel_enum)
  Constant34/1 -> Min6/2
  Min6/1 -> RollingAverage5/1(KVMC_RollAveLevel_enum)

== system vmc/VMC/VMC/Long Acceleration Calculation/Vehicle to Meter Speed ==
  InputSpeed : Inport
  Add4 : Sum
  Constant16 : Constant  Value=KVMC_Veh2MeterSpdFactor_enum
  Constant23 : Constant  Value=KVMC_Veh2MeterSpdOffset_enum
  Constant28 : Constant  Value=KVMC_Veh2MeterSpdLoFactor_enum
  Divide5 : Product  Inputs=**
  Divide8 : Product  Inputs=**
  Switch : Switch  Criteria=u2 > Threshold  Threshold=KVMC_Veh2MeterSpdLoBdy_kph
  OutputSpeed : Outport
  wires:
  Add4/1 -> Switch/1
  Divide5/1 -> Add4/2
  Constant16/1 -> Divide5/1
  InputSpeed/1 -> Divide5/2, Switch/2, Divide8/1
  Constant23/1 -> Add4/1
  Constant28/1 -> Divide8/2
  Divide8/1 -> Switch/3
  Switch/1 -> OutputSpeed/1

== system vmc/VMC/VMC/MSA function/Anti-Speed Limitation ==
  VINP_HoodSW_flg : Inport
  VTQD_GearActualPosn_enum : Inport  Port=2
  VINP_SmartEcoModeSW_flg : Inport  Port=3
  VVMC_APSActive_flg : Inport  Port=4
  VVMC_IntMSACtrlSta_enum : Inport  Port=5
  AND : Logic  Inputs=3  AllPortsSameDT=off  OutDataTypeStr=boolean
  AND1 : Logic  AllPortsSameDT=off  OutDataTypeStr=boolean
  AND2 : Logic  Inputs=3  AllPortsSameDT=off  OutDataTypeStr=boolean
  AND3 : Logic  AllPortsSameDT=off  OutDataTypeStr=boolean
  AND4 : Logic  Inputs=3  AllPortsSameDT=off  OutDataTypeStr=boolean
  Constant1 : Constant  Value=KVMC_AntiSpdLimSW_flg
  Constant2 : Constant  Value=ENUM_GEARACTUALPOSN_D
  Constant3 : Constant  Value=KVMC_SmartEcoPlusSW_flg
  Constant4 : Constant  Value=ENUM_GEARACTUALPOSN_D
  Constant5 : Constant  Value=KVMC_AntiSpdLim_kph
  Constant6 : Constant  Value=KVMC_SmartEcoLimitSpd_kph
  Constant7 : Constant  Value=ENUM_ADASMSASTA_ACTIVE
  Constant8 : Constant  Value=ENUM_ADASMSASTA_ACTIVE
  Constant9 : Constant  Value=ENUM_ADASMSASTA_STANDBY
  Equal : RelationalOperator  Operator===  OutDataTypeStr=boolean  RndMeth=Simplest
  Equal1 : RelationalOperator  Operator===  OutDataTypeStr=boolean  RndMeth=Simplest
  Equal2 : RelationalOperator  Operator=~=  OutDataTypeStr=boolean  RndMeth=Simplest
  Equal3 : RelationalOperator  Operator=~=  OutDataTypeStr=boolean  RndMeth=Simplest
  Equal4 : RelationalOperator  Operator=~=  OutDataTypeStr=boolean  RndMeth=Simplest
  NOT : Logic  Operator=NOT  AllPortsSameDT=off  OutDataTypeStr=boolean
  OR : Logic  Operator=OR  AllPortsSameDT=off  OutDataTypeStr=boolean
  OR1 : Logic  Operator=OR  AllPortsSameDT=off  OutDataTypeStr=boolean
  OR2 : Logic  Operator=OR  AllPortsSameDT=off  OutDataTypeStr=boolean
  Switch : Switch  Criteria=u2 > Threshold
  VVMC_AntiSpdLimEn_flg : Outport
  VVMC_AntiLimitSpd_kph : Outport  Port=2
  VVMC_AntiSpdLimSpdEn_flg : Outport  Port=3
  VVMC_AntiSpdLimStaEn_flg : Outport  Port=4
  wires:
  VINP_HoodSW_flg/1 -> [VINP_HoodSW_flg]
  VTQD_GearActualPosn_enum/1 -> [VTQD_GearActualPosn_enum]
  VVMC_IntMSACtrlSta_enum/1 -> [VVMC_IntMSACtrlSta_enum]
  VVMC_APSActive_flg/1 -> [VVMC_APSActive_flg]
  VINP_SmartEcoModeSW_flg/1 -> [VINP_SmartEcoModeSW_flg]
  OR/1 -> [VVMC_AntiSpdLimEn_flg]  "VVMC_AntiSpdLimEn_flg"
  Constant7/1 -> Equal2/2
  [VINP_HoodSW_flg] -> AND/1
  OR1/1 -> [VVMC_AntiSpdLimSpdEn_flg]  "VVMC_AntiSpdLimSpdEn_flg"
  [VVMC_HoodSpdLimitEn_flg] -> Switch/2
  OR2/1 -> [VVMC_AntiSpdLimStaEn_flg]  "VVMC_AntiSpdLimStaEn_flg"
  Constant1/1 -> AND/3
  [VVMC_HoodSpdLimitEn_flg] -> OR1/2
  AND3/1 -> OR1/1
  AND4/1 -> OR2/1
  Equal1/1 -> AND2/2
  Equal4/1 -> AND4/3
  [VVMC_HoodSpdLimitEn_flg] -> OR2/2
  [VVMC_APSActive_flg] -> NOT/1
  Constant9/1 -> Equal4/2
  [VVMC_AntiSpdLimEn_flg] -> AND4/1
  [VVMC_IntMSACtrlSta_enum] -> Equal2/1
  [VVMC_SmartEcoEn_flg] -> OR/2
  Constant8/1 -> Equal3/2
  Equal3/1 -> AND4/2
  AND/1 -> [VVMC_HoodSpdLimitEn_flg]  "VVMC_HoodSpdLimitEn_flg"
  [VVMC_IntMSACtrlSta_enum] -> Equal3/1
  Switch/1 -> [VVMC_AntiLimitSpd_kph]  "VVMC_AntiLimitSpd_kph"
  [VVMC_IntMSACtrlSta_enum] -> Equal4/1
  [VVMC_AntiSpdLimEn_flg] -> AND3/1
  Equal/1 -> AND/2
  Constant3/1 -> AND1/2
  Equal2/1 -> AND3/2
  AND1/1 -> AND2/1
  [VINP_SmartEcoModeSW_flg] -> AND1/1
  [VVMC_HoodSpdLimitEn_flg] -> OR/1
  Constant5/1 -> Switch/1
  AND2/1 -> [VVMC_SmartEcoEn_flg]  "VVMC_SmartEcoEn_flg"
  Constant4/1 -> Equal1/2
  Constant2/1 -> Equal/2
  [VTQD_GearActualPosn_enum] -> Equal/1
  NOT/1 -> AND2/3
  Constant6/1 -> Switch/3
  [VTQD_GearActualPosn_enum] -> Equal1/1
  [VVMC_AntiSpdLimStaEn_flg] -> VVMC_AntiSpdLimStaEn_flg/1
  [VVMC_AntiSpdLimEn_flg] -> VVMC_AntiSpdLimEn_flg/1
  [VVMC_AntiSpdLimSpdEn_flg] -> VVMC_AntiSpdLimSpdEn_flg/1
  [VVMC_AntiLimitSpd_kph] -> VVMC_AntiLimitSpd_kph/1
